simulink model "Hito1"  (R2023b)
settings: Solver=FixedStepAuto  StartTime=0.0  StopTime=inf  RelTol=1e-3  EnableMultiTasking=on
libraries: simulink x8
settings Model: ExtModeTrigDuration=2  Creator=mmgac  LastModifiedBy=jaime
settings SolverCC: AutoInsertRateTranBlk=on
settings OptimizationCC: EnhancedBackFolding=on  PassReuseOutputArgsThreshold=0  MaxStackSize=64  OptimizeBlockOrder=speed  DifferentSizesBufferReuse=on  OptimizationCustomize=off
settings DebuggingCC: ParameterTunabilityLossMsg=error
settings HardwareCC: ProdBitPerInt=16  ProdBitPerPointer=16  ProdBitPerSizeT=16  ProdBitPerPtrDiffT=16  ProdLargestAtomicFloat=None  ProdWordSize=8  ProdHWDeviceType=Atmel->AVR  UseEmbeddedCoderFeatures=off  UseSimulinkCoderFeatures=off
settings SFSimCC: MATLABDynamicMemAlloc=off
settings RTWCC: Description=Embedded Coder  SystemTargetFile=ert.tlc  HardwareBoard=Arduino Mega 2560  TemplateMakefile=ert_default_tmf  Toolchain=Arduino AVR  BuildConfiguration=Faster Runs
settings CodeAppCC: ForceParamTrailComments=on  OperatorAnnotations=on  MangleLength=10
settings ERTTargetCC: ERTCustomFileBanners=off  SupportContinuousTime=on  SupportNonInlinedSFcns=on  RemoveResetFunc=off  SupportVariableSizeSignals=on  ModelStepFunctionPrototypeControlCompliant=off  ExtModeTransport=3  ExtModeStaticAlloc=on  ExtModeAutomaticAllocSize=off  ExtModeStaticAllocSize=2048  ExtModeMexFile=ext_xcp  ExtModeIntrfLevel=Level2 - Open

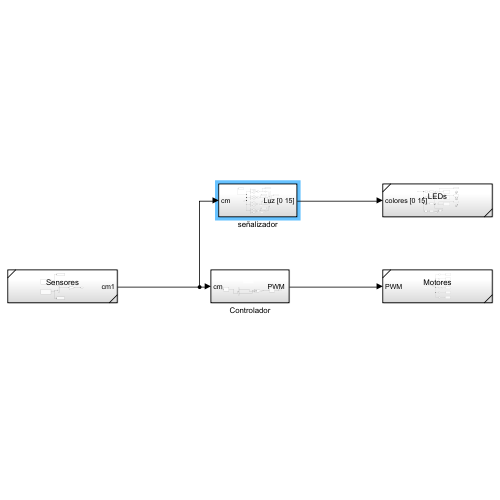
[thumbnail: Simulink's stored preview of the top-level diagram]
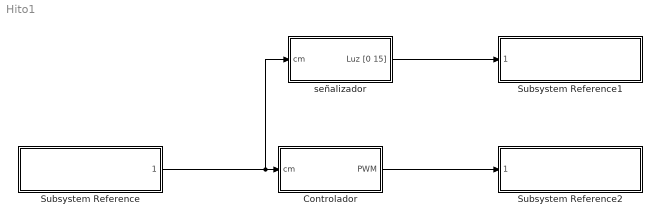
== system Hito1 ==
  Controlador : Subsystem
  Subsystem Reference : Subsystem  ReferencedSubsystem=Sensores
  Subsystem Reference1 : Subsystem  ReferencedSubsystem=LEDs
  Subsystem Reference2 : Subsystem  ReferencedSubsystem=Motores
  señalizador : Subsystem
  wires:
  Controlador/1("PWM ") -> Subsystem Reference2/1
  señalizador/1(Luz [0 15]) -> Subsystem Reference1/1
  Subsystem Reference/1 -> señalizador/1(cm), Controlador/1(cm)

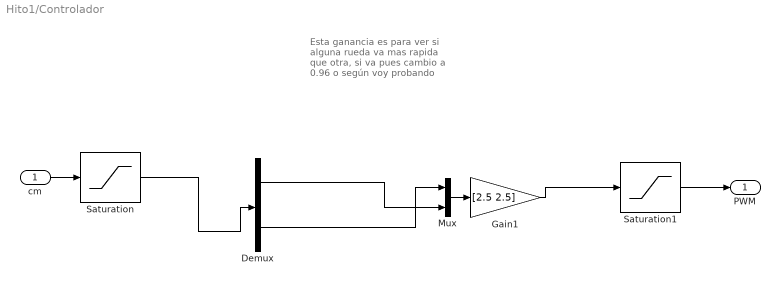
== system Hito1/Controlador ==
  note: Esta ganancia es para ver si alguna rueda va mas rapida que otra, si va pues cambio a 0.96 o según voy probando
  cm : Inport
  Demux : Demux  Outputs=2
  Gain1 : Gain  Gain=[2.5 2.5]  OutDataTypeStr=int16
  Mux : Mux  Inputs=2
  Saturation : Saturate  UpperLimit=100  LowerLimit=9
  Saturation1 : Saturate  UpperLimit=100  LowerLimit=9
  "PWM " : Outport
  wires:
  cm/1 -> Saturation/1
  Mux/1 -> Gain1/1
  Saturation/1 -> Demux/1
  Demux/1 -> Mux/2
  Demux/2 -> Mux/1
  Gain1/1 -> Saturation1/1
  Saturation1/1 -> "PWM "/1

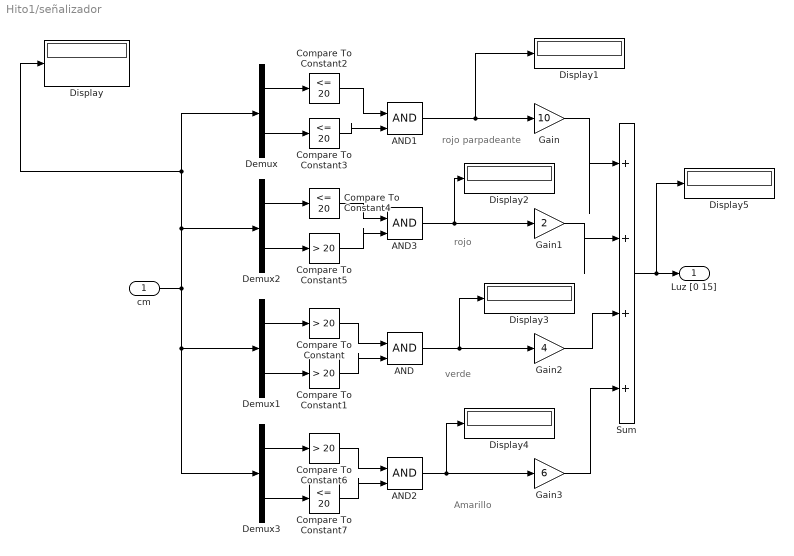
== system Hito1/señalizador ==
  note: verde
  note: rojo
  note: rojo parpadeante
  note: Amarillo
  cm : Inport
  AND{,1..3} (4 alike) : Logic  IconShape=distinctive  AllPortsSameDT=off  OutDataTypeStr=boolean
  Compare To Constant{,1,5..6} (4 alike) : simulink/Logic and Bit Operations/Compare To Constant  relop=>  const=20  OutDataTypeStr=boolean
  Compare To Constant{2..4,7} (4 alike) : simulink/Logic and Bit Operations/Compare To Constant  relop=<=  const=20  OutDataTypeStr=boolean
  Demux{,1..3} (4 alike) : Demux  Outputs=2
  Display{,1..5} (6 alike) : Display
  Gain : Gain  Gain=10
  Gain1 : Gain  Gain=2
  Gain2 : Gain  Gain=4
  Gain3 : Gain  Gain=6
  Sum : Sum  Inputs=|++++  OutDataTypeStr=int16
  Luz [0 15] : Outport
  wires:
  cm/1 -> Display/1, Demux/1, Demux2/1, Demux3/1, Demux1/1
  Demux1/1 -> Compare To Constant/1
  Demux1/2 -> Compare To Constant1/1
  Compare To Constant/1 -> AND/1
  Compare To Constant1/1 -> AND/2
  Demux/1 -> Compare To Constant2/1
  Demux/2 -> Compare To Constant3/1
  Demux2/2 -> Compare To Constant5/1
  Demux2/1 -> Compare To Constant4/1
  Compare To Constant2/1 -> AND1/1
  Compare To Constant3/1 -> AND1/2
  Demux3/2 -> Compare To Constant7/1
  Compare To Constant6/1 -> AND2/1
  Compare To Constant7/1 -> AND2/2
  Demux3/1 -> Compare To Constant6/1
  Compare To Constant4/1 -> AND3/1
  Compare To Constant5/1 -> AND3/2
  AND3/1 -> Display2/1, Gain1/1
  AND1/1 -> Display1/1, Gain/1
  AND2/1 -> Display4/1, Gain3/1
  Gain/1 -> Sum/1
  Gain1/1 -> Sum/2
  Gain2/1 -> Sum/3
  Gain3/1 -> Sum/4
  AND/1 -> Display3/1, Gain2/1
  Sum/1 -> Display5/1, Luz [0 15]/1
